simulink model "Sprott"  (R2017a)
settings: Solver=VariableStepAuto  StartTime=0.0  StopTime=20  FixedStep=1  RelTol=1e-3  SampleTimeConstraint=STIndependent  EnableMultiTasking=on
libraries: dspvision x1, simulink x1
settings Model: Creator=Luis  LastModifiedBy=Radian
settings DataIOCC: MaxDataPoints=10000000  SaveFormat=Array
settings OptimizationCC: LifeSpan=inf
settings DebuggingCC: SolverPrmCheckMsg=warning  SFUnexpectedBacktrackingDiag=warning  SFNoUnconditionalDefaultTransitionDiag=warning  SFExecutionAtInitializationDiag=none
settings HardwareCC: ProdBitPerPointer=32  ProdBitPerSizeT=32  ProdBitPerPtrDiffT=32  ProdLargestAtomicFloat=None  ProdIntDivRoundTo=Undefined  ProdEndianess=Unspecified  ProdWordSize=32  ProdHWDeviceType=32-bit Generic
settings ModelReferenceCC: PropagateSignalLabelsOutOfModel=off
settings GRTTargetCC: TargetLangStandard=C89/C90 (ANSI)  GeneratePreprocessorConditionals=Disable all
settings ConfigComp: CovMetricSettings=dw  CovHtmlReporting=on  CovSaveCumulativeToWorkspaceVar=on  CovSaveSingleToWorkspaceVar=on  CovExternalEMLEnable=off  CovSFcnEnable=off

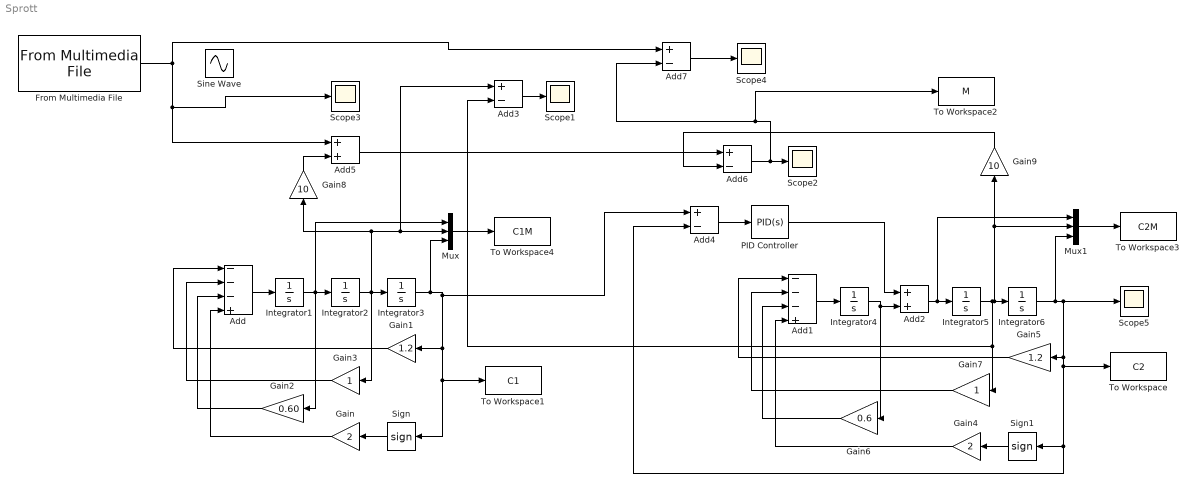
== system Sprott ==
  Add : Sum  Inputs=---+
  Add1 : Sum  Inputs=---+
  Add2 : Sum
  Add{3..4,6..7} (4 alike) : Sum  Inputs=+-
  Add5 : Sum
  From Multimedia File : dspvision/From Multimedia File  inputFilename=speech_dft.mp3  loop=on  numPlays=inf  outputStreams=Audio only  videoDataType=single  audioDataType=double  inheritSampleTime=on  userDefinedSampleTime=1/30  noAudioOutput=off  isIntensityVideo=off  fourcc=RGB  colorVideoFormat=Separate color signals  outputEOF=off  dataOrg=Column-major  audioFrameSize=1  computeAudioFrameSize=off  outSamplingMode=Frame based
      settings: SourceProductBaseCode=VP
  Gain : Gain  Gain=2
  Gain1 : Gain  Gain=1.2
  Gain2 : Gain  Gain=0.60
  Gain3 : Gain
  Gain4 : Gain  Gain=2
  Gain5 : Gain  Gain=1.2
  Gain6 : Gain  Gain=0.6
  Gain7 : Gain
  Gain8 : Gain  Gain=10
  Gain9 : Gain  Gain=10
  Integrator1 : Integrator  InitialCondition=1.1
  Integrator2 : Integrator
  Integrator3 : Integrator  InitialCondition=-1
  Integrator4 : Integrator  InitialCondition=0.1
  Integrator5 : Integrator  InitialCondition=0.1
  Integrator6 : Integrator  InitialCondition=0.1
  Mux : Mux  Inputs=3
  Mux1 : Mux  Inputs=3
  PID Controller : simulink/Continuous/PID Controller  Controller=PID  TimeDomain=Continuous-time  SampleTime=-1  IntegratorMethod=Forward Euler  FilterMethod=Forward Euler  Form=Parallel  UseFilter=on  ControllerParametersSource=internal  P=4  I=0.5  D=2  N=381.341034168083  InitialConditionSource=internal  InitialConditionForIntegrator=0  InitialConditionForFilter=0  ExternalReset=none  LimitOutput=off  UpperSaturationLimit=inf  LowerSaturationLimit=-inf  LinearizeAsGain=on  AntiWindupMode=none  Kb=1  TrackingMode=off  Kt=1  PParamMin=[]  PParamMax=[]  IParamMin=[]  IParamMax=[]  DParamMin=[]  DParamMax=[]  NParamMin=[]  NParamMax=[]  KbParamMin=[]  KbParamMax=[]  KtParamMin=[]  KtParamMax=[]  POutMin=[]  POutMax=[]  IOutMin=[]  IOutMax=[]  DOutMin=[]  DOutMax=[]  NOutMin=[]  NOutMax=[]  KbOutMin=[]  KbOutMax=[]  KtOutMin=[]  KtOutMax=[]  IntegratorOutMin=[]  IntegratorOutMax=[]  FilterOutMin=[]  FilterOutMax=[]  SumOutMin=[]  SumOutMax=[]  SumI1OutMin=[]  SumI1OutMax=[]  SumI2OutMin=[]  SumI2OutMax=[]  SumI3OutMin=[]  SumI3OutMax=[]  SumDOutMin=[]  SumDOutMax=[]  SaturationOutMin=[]  SaturationOutMax=[]  IntegratorContinuousStateAttributes=''  IntegratorStateMustResolveToSignalObject=off  IntegratorRTWStateStorageClass=Auto  FilterContinuousStateAttributes=''  FilterStateMustResolveToSignalObject=off  FilterRTWStateStorageClass=Auto  DifferentiatorICPrevScaledInput=0  DifferentiatorOutMin=[]  DifferentiatorOutMax=[]  InitialConditionSetting=State (most efficient)
  Scope{1..5} (5 alike) : Scope
  Sign : Signum
  Sign1 : Signum
  Sine Wave : Sin  Amplitude=.5  Frequency=3000  SampleTime=1/44100
  To Workspace : ToWorkspace  VariableName=C2  SaveFormat=Structure With Time  SampleTime=-1
  To Workspace1 : ToWorkspace  VariableName=C1  SaveFormat=Structure With Time  SampleTime=-1
  To Workspace2 : ToWorkspace  VariableName=M  SaveFormat=Structure With Time  SampleTime=-1
  To Workspace3 : ToWorkspace  VariableName=C2M  SaveFormat=Structure With Time  SampleTime=-1
  To Workspace4 : ToWorkspace  VariableName=C1M  SaveFormat=Structure With Time  SampleTime=-1
  wires:
  Integrator1/1 -> Integrator2/1, Gain2/1, Mux/1
  Integrator2/1 -> Mux/2, Add3/1, Gain8/1, Gain3/1, Integrator3/1
  Sign/1 -> Gain/1
  Gain/1 -> Add/4
  Gain2/1 -> Add/3
  Integrator3/1 -> Add4/1, Sign/1, To Workspace1/1, Gain1/1, Mux/3
  Gain1/1 -> Add/1
  Gain3/1 -> Add/2
  Add/1 -> Integrator1/1
  Integrator4/1 -> Add2/2, Gain6/1
  Integrator5/1 -> Gain9/1, Mux1/2, Integrator6/1, Add3/2, Gain7/1
  Sign1/1 -> Gain4/1
  Gain4/1 -> Add1/4
  Gain6/1 -> Add1/3
  Integrator6/1 -> Mux1/3, Scope5/1, Add4/2, Sign1/1, To Workspace/1, Gain5/1
  Gain5/1 -> Add1/1
  Gain7/1 -> Add1/2
  Add1/1 -> Integrator4/1
  Add2/1 -> Mux1/1, Integrator5/1
  Add4/1 -> PID Controller/1
  PID Controller/1 -> Add2/1
  Gain8/1 -> Add5/2
  Add5/1 -> Add6/1
  Gain9/1 -> Add6/2
  Mux/1 -> To Workspace4/1
  Add6/1 -> Add7/2, To Workspace2/1, Scope2/1
  Add3/1 -> Scope1/1
  Add7/1 -> Scope4/1
  Mux1/1 -> To Workspace3/1
  From Multimedia File/1 -> Scope3/1, Add5/1, Add7/1
